simulink library "ConfigHandler"  (R2016b)
settings: Solver=VariableStepAuto  StartTime=0.0  StopTime=10.0  RelTol=1e-3
undefined symbols (not defined in the file or in its folder): resolutionJointEncoder, sampleTimeSimulink
libraries: ConversionsLibrary x4
settings Model: Creator=Nathan  LastModifiedBy=march

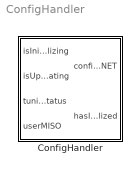
== system ConfigHandler ==
  ConfigHandler : Subsystem

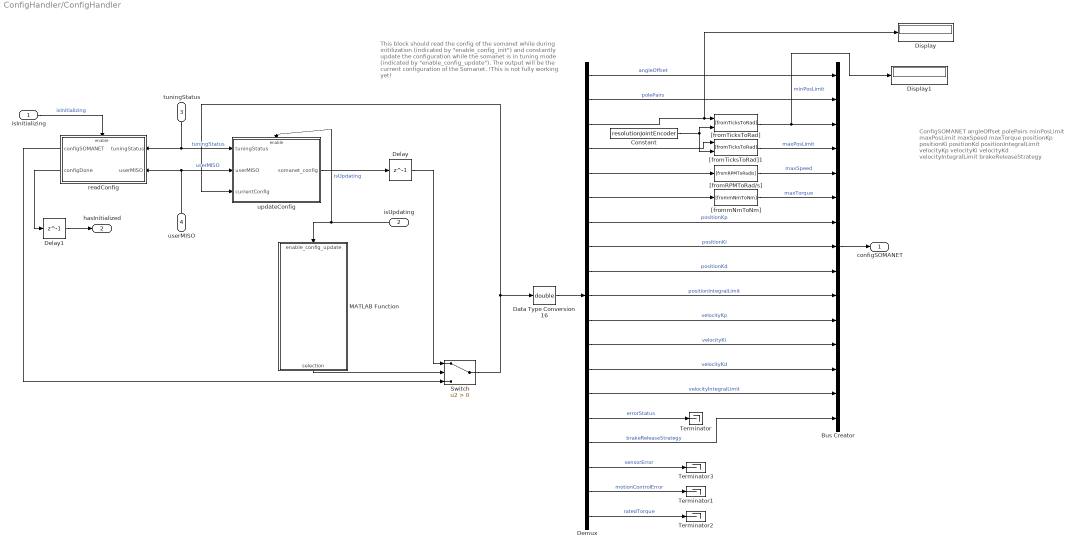
== system ConfigHandler/ConfigHandler ==
  note: This block should read the config of the somanet while
      | during initilization (indicated by "enable_config_init") and
      | constantly update the configuration while the somanet
      | is in tuning mode (indicated by "enable_config_update").
      | The output will be the current configuration of the Somanet.
      | !This is not fully working yet!
  note: ConfigSOMANET
      | angleOffset
      | polePairs
      | minPosLimit
      | maxPosLimit
      | maxSpeed
      | maxTorque
      | positionKp
      | positionKi
      | positionKd
      | positionIntegralLimit
      | velocityKp
      | velocityKi
      | velocityKd
      | velocityIntegralLimit
      | brakeReleaseStrategy
  isInitializing : Inport  PortDimensions=1  SampleTime=[0.002,0]
  isUpdating : Inport  Port=2  PortDimensions=1  SampleTime=[0.002,0]
  tuningStatus : Inport  Port=3  PortDimensions=1  SampleTime=[0.002,0]
  userMISO : Inport  Port=4  PortDimensions=1  SampleTime=[0.002,0]
  Bus Creator : BusCreator  Inputs=15  OutDataTypeStr=Bus: JointControlConfig  NonVirtualBus=on
  Constant : Constant  Value=resolutionJointEncoder
  Data Type Conversion16 : DataTypeConversion  OutDataTypeStr=double
  Delay : Delay  DelayLength=1
  Delay1 : Delay  DelayLength=1
  Demux : Demux  Outputs=19
  Display : Display
  Display1 : Display
  MATLAB Function : MATLAB Function  TreatAsAtomicUnit=on  SystemSampleTime=sampleTimeSimulink
  Switch : Switch  Criteria=u2 > Threshold
  Terminator{,1..3} (4 alike) : Terminator
  "[fromRPMToRad/s]" : ConversionsLibrary/[fromRPMToRad//s]
  "[fromTicksToRad]" : ConversionsLibrary/[fromTicksToRad]
  "[fromTicksToRad]1" : ConversionsLibrary/[fromTicksToRad]
  "[frommNmToNm]" : ConversionsLibrary/[frommNmToNm]
  readConfig : Subsystem  TreatAsAtomicUnit=on
  updateConfig : Subsystem  TreatAsAtomicUnit=on
  configSOMANET : Outport  OutDataTypeStr=Bus: JointControlConfig  BusOutputAsStruct=on
  hasInitialized : Outport  Port=2  PortDimensions=1  SampleTime=[0.002,0]
  wires:
  Data Type Conversion16/1 -> Demux/1
  Demux/6 -> "[frommNmToNm]"/1
  Demux/5 -> "[fromRPMToRad/s]"/1
  Demux/4 -> "[fromTicksToRad]1"/1
  Demux/3 -> "[fromTicksToRad]"/1, Display/1
  Switch/1 -> updateConfig/3(currentConfig), Data Type Conversion16/1
  Constant/1 -> "[fromTicksToRad]"/2, "[fromTicksToRad]1"/2
  Demux/16 -> Bus Creator/15  "brakeReleaseStrategy"
  Demux/14 -> Bus Creator/14  "velocityIntegralLimit"
  Demux/13 -> Bus Creator/13  "velocityKd"
  Demux/12 -> Bus Creator/12  "velocityKi"
  Demux/11 -> Bus Creator/11  "velocityKp"
  Demux/10 -> Bus Creator/10  "positionIntegralLimit"
  Demux/9 -> Bus Creator/9  "positionKd"
  Demux/8 -> Bus Creator/8  "positionKi"
  Demux/7 -> Bus Creator/7  "positionKp"
  Demux/2 -> Bus Creator/2  "polePairs"
  Demux/1 -> Bus Creator/1  "angleOffset"
  "[frommNmToNm]"/1 -> Bus Creator/6  "maxTorque"
  "[fromTicksToRad]1"/1 -> Bus Creator/4  "maxPosLimit"
  "[fromTicksToRad]"/1 -> Bus Creator/3, Display1/1  "minPosLimit"
  "[fromRPMToRad/s]"/1 -> Bus Creator/5  "maxSpeed"
  updateConfig/1(somanet_config) -> Delay/1
  tuningStatus/1 -> updateConfig/1(tuningStatus), readConfig/1(tuningStatus)  "tuningStatus"
  userMISO/1 -> updateConfig/2(userMISO), readConfig/2(userMISO)  "userMISO"
  readConfig/2(configDone) -> Delay1/1
  isInitializing/1 -> readConfig/Enable  "isInitializing"
  Delay1/1 -> hasInitialized/1
  readConfig/1(configSOMANET) -> Switch/3
  Delay/1 -> Switch/1
  Bus Creator/1 -> configSOMANET/1
  MATLAB Function/1(selection) -> Switch/2
  Demux/18 -> Terminator1/1  "motionControlError"
  isUpdating/1 -> updateConfig/Enable, MATLAB Function/1(enable_config_update)  "isUpdating"
  Demux/15 -> Terminator/1  "errorStatus"
  Demux/17 -> Terminator3/1  "sensorError"
  Demux/19 -> Terminator2/1  "ratedTorque"

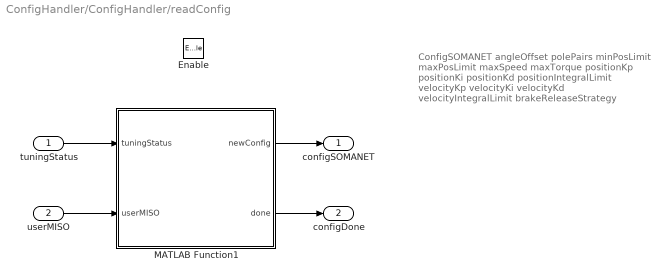
== system ConfigHandler/ConfigHandler/readConfig ==
  note: ConfigSOMANET
      | angleOffset
      | polePairs
      | minPosLimit
      | maxPosLimit
      | maxSpeed
      | maxTorque
      | positionKp
      | positionKi
      | positionKd
      | positionIntegralLimit
      | velocityKp
      | velocityKi
      | velocityKd
      | velocityIntegralLimit
      | brakeReleaseStrategy
  tuningStatus : Inport
  userMISO : Inport  Port=2
  Enable : EnablePort
  MATLAB Function1 : MATLAB Function  TreatAsAtomicUnit=on  SystemSampleTime=sampleTimeSimulink
  configSOMANET : Outport
  configDone : Outport  Port=2
  wires:
  userMISO/1 -> MATLAB Function1/2(userMISO)
  tuningStatus/1 -> MATLAB Function1/1(tuningStatus)
  MATLAB Function1/2(done) -> configDone/1
  MATLAB Function1/1(newConfig) -> configSOMANET/1

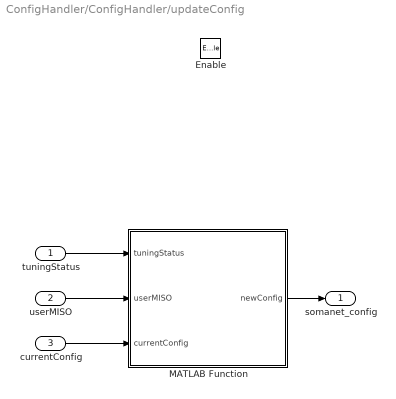
== system ConfigHandler/ConfigHandler/updateConfig ==
  tuningStatus : Inport
  userMISO : Inport  Port=2
  currentConfig : Inport  Port=3
  Enable : EnablePort
  MATLAB Function : MATLAB Function  TreatAsAtomicUnit=on  SystemSampleTime=sampleTimeSimulink
  somanet_config : Outport
  wires:
  userMISO/1 -> MATLAB Function/2(userMISO)
  MATLAB Function/1(newConfig) -> somanet_config/1
  currentConfig/1 -> MATLAB Function/3(currentConfig)
  tuningStatus/1 -> MATLAB Function/1(tuningStatus)

== matlab function ConfigHandler/MATLAB Function ==
  data: enable_config_update input; selection output
function selection = select_config_loop(enable_config_update)
%% Selects whether to output values from read_config or from update_config
% Once update_config has run once, that config stores the correct values
% So, after going back to cyclic operation from tuning mode, update_config
% outputs the correct config even though it's not running
% Therefore: if enable_config_update was true ever, always pick the values
% from update_config

persistent post_init;
if isempty(post_init)
    post_init = false;
end
post_init = or(post_init, enable_config_update);
selection = post_init;
end

== matlab function ConfigHandler/readConfig/MATLAB Function1 ==
  data: tuningStatus input; newConfig output int32; userMISO input; done output
function [newConfig,done] = read_config(tuningStatus,userMISO)
    persistent calls;
    persistent buffered_config;
    N_params = 19;
    if(isempty(calls))
        calls = 0;
        buffered_config = zeros(N_params,1);
    end
  
    
    status_mux = bitand(bitsra(tuningStatus,16),hex2dec('FF'));
   
    if status_mux <= N_params && status_mux >= 1
        calls = calls + 1;
        buffered_config(status_mux) = userMISO;
        %TODO error handling here?
    end
    
    if calls > N_params + 10 % we might want to increase this. We have noticed that sometimes an important value like maxpos does not get properly initalized and instead is zero
        done = true;
    else
        done = false;
    end
    
    newConfig = to_signed_int32(buffered_config);
end

== matlab function ConfigHandler/updateConfig/MATLAB Function ==
  data: tuningStatus input; newConfig output; userMISO input; currentConfig input
function newConfig = update_config(tuningStatus,userMISO,currentConfig)
    status_mux = bitand(bitsra(tuningStatus,16),hex2dec('FF'));
    N_params = 19;
    
    newConfig = currentConfig;
    if status_mux <= N_params
        newConfig(status_mux) = to_signed_int32(userMISO);
        %TODO error handling here?
    end
